simulink model "ad9361_qpsk_test"  (R2019a)
settings: Solver=ode23  StartTime=0.0  StopTime=inf  RelTol=1e-3  EnableMultiTasking=on
undefined symbols (not defined in the file or in its folder): doppler, magnitude
libraries: simulink x11, commdigbbndpm3 x10, dspmathops x4, commrandsrc3 x4, commseqgen3 x4, commfilt2 x3, ad9371_utilities x2, commutil2 x2, ad9361_models x2, commsink2 x1, commchan3 x1, commcnvcod2 x1
settings Model: SimulationMode=accelerator  NumberOfSteps=100  Creator=The MathWorks Inc.  LastModifiedBy=Terasoft
settings SolverCC: MinimalZcImpactIntegration=on
settings DataIOCC: ExternalInput=txWaveform  SaveFormat=StructureWithTime  SaveOutput=off  SignalLogging=off  DSMLogging=off  SaveTime=off  ReturnWorkspaceOutputs=off  OutputSaveName=rx
settings OptimizationCC: DefaultParameterBehavior=Inlined  InlineInvariantSignals=on  EfficientMapNaN2IntZero=off  LifeSpan=inf  SimCompilerOptimization=on
settings DebuggingCC: ReadBeforeWriteMsg=DisableAll  WriteAfterWriteMsg=DisableAll  WriteAfterReadMsg=DisableAll  UnderspecifiedInitializationDetection=Classic  MergeDetectMultiDrivingBlocksExec=none  SolverPrmCheckMsg=warning  InheritedTsInSrcMsg=none  MultiTaskDSMMsg=none  IntegerOverflowMsg=none  AllowSymbolicDim=off  PregeneratedLibrarySubsystemCodeDiagnostic=none  SFUnexpectedBacktrackingDiag=warning  SFNoUnconditionalDefaultTransitionDiag=none  SFUndirectedBroadcastEventsDiag=none  SFExecutionAtInitializationDiag=none  IntegerSaturationMsg=none  ArithmeticOperatorsInVariantConditions=warning
settings HardwareCC: ProdBitPerPointer=32  ProdBitPerSizeT=32  ProdBitPerPtrDiffT=32  ProdLargestAtomicFloat=None  ProdIntDivRoundTo=Undefined  ProdEndianess=Unspecified  ProdWordSize=32  ProdHWDeviceType=32-bit Generic  TargetBitPerPointer=64  TargetBitPerSizeT=64  TargetBitPerPtrDiffT=64  TargetLongLongMode=on  TargetIntDivRoundTo=Zero  TargetEndianess=LittleEndian  TargetWordSize=64  TargetHWDeviceType=MATLAB Host  ProdEqTarget=off
settings ModelReferenceCC: UpdateModelReferenceTargets=IfOutOfDate  PropagateSignalLabelsOutOfModel=off
settings SFSimCC: SFSimEcho=off  SimUseLocalCustomCode=off
settings RTWCC: RTWUseLocalCustomCode=off
settings CodeAppCC: MaxIdLength=128
settings GRTTargetCC: TargetLangStandard=C89/C90 (ANSI)  CombineOutputUpdateFcns=off  GRTInterface=on
settings ConfigComp: CovMetricSettings=dw  CovHtmlReporting=on  CovSaveCumulativeToWorkspaceVar=on  CovSaveSingleToWorkspaceVar=on  CovExternalEMLEnable=off  CovSFcnEnable=off
settings SimscapeCC: ExplicitSolverDiagnosticOptions=none  SimscapeNormalizeSystem=off

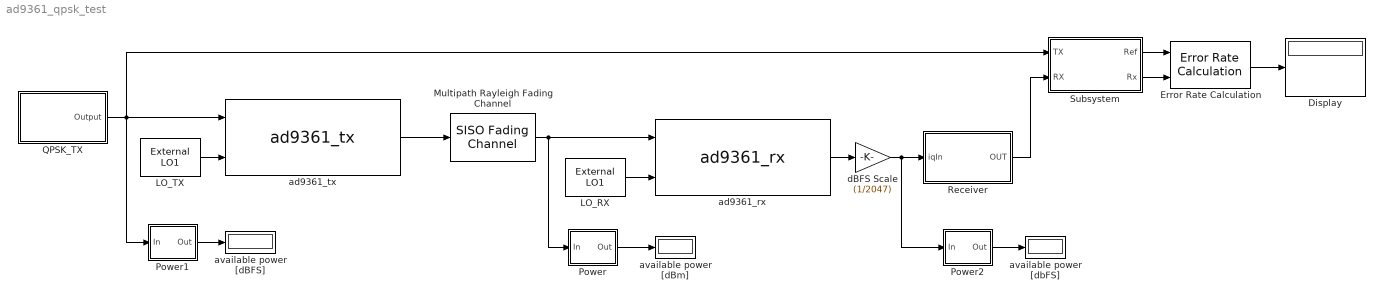
== system ad9361_qpsk_test ==
  Display : Display
  Error Rate Calculation : commsink2/Error Rate Calculation  N=21  st_delay=525  cp_mode=Entire frame  subframe=[]  PMode=Port  WsName=ErrorVec  RsMode2=off  stop=off  numErr=100  maxBits=1e6
      settings: SourceProductName=Communications Toolbox
  LO_RX : ad9371_utilities/External LO1  PN=[-95 -110 -110 -125 -157]  Freq=[1e3 1e4 1e5 1e6 3e6]  PH=Random
      settings: SourceProductName=RF Blockset Models for Analog Devices RF Transceivers  SourceProductBaseCode=SIM_RF_TRANS
  LO_TX : ad9371_utilities/External LO1  PN=[-95 -110 -110 -125 -157]  Freq=[1e3 1e4 1e5 1e6 3e6]  PH=Random
      settings: SourceProductName=RF Blockset Models for Analog Devices RF Transceivers  SourceProductBaseCode=SIM_RF_TRANS
  Multipath Rayleigh Fading Channel : commchan3/SISO Fading Channel  InheritSampleRate=off  SampleRate=122.88e6  PathDelays=[0 3e-8 5e-7]  AveragePathGains=[0 -15 -30]-60 %[0 -15 -30]-40  NormalizePathGains=off  FadingDistribution=Rayleigh  KFactor=3  DirectPathDopplerShift=0  DirectPathInitialPhase=0  MaximumDopplerShift=25  DopplerSpectrum=doppler('Jakes')  ChannelInterpolationMethod=Polyphase  RandomStream=mt19937ar with seed  RandomNumGenerator=shr3cong  Seed=54873  PathGainsOutputPort=off  ChannelFilterDelayOutputPort=off  SimulateUsing=Code generation  Visualization=Off  PathsForDopplerDisplay=1  SamplesToDisplay=25%
      settings: SourceProductName=Communications Toolbox
  Power : Subsystem  mask{R=1}
      mask prompts: R "Reference Impedance [Ohm]"
      mask DialogControl DescGroupVar Prompt: Power Meter
      mask Display: disp('Power \nMeter');
  Power1 : Subsystem  mask{R=1}
      mask prompts: R "Reference Impedance [Ohm]"
      mask DialogControl DescGroupVar Prompt: Power Meter
      mask Display: disp('Power \nMeter');
  Power2 : Subsystem  mask{R=1}
      mask prompts: R "Reference Impedance [Ohm]"
      mask DialogControl DescGroupVar Prompt: Power Meter
      mask Display: disp('Power \nMeter');
  QPSK_TX : Subsystem  mask{Rs=7.68e6, N=4}
      mask prompts: Rs "Sample Rate (Hz)"; N "Samples Per Symbol"
      mask init:
      | PadStart = 100;
      | PadEnd = 100;
      | HeaderBitLength = 16;
      | AGCSequence = 16;
      | AGCPreambleLength = 160;
      | TimingPreambleLength = 28;
      | DFEDataLength = 250;
      | PayloadBitLength = 156;
      | modulatedSymbols = 250;
      | bitsPerSample = 2;
      | 
      | FrameLength = PadStart + AGCPreambleLength + TimingPreambleLength + DFEDataLength + HeaderBitLength + PayloadBitLength + PadEnd;
      | FramePeriod = (FrameLength*N)/Rs;
      mask Display: disp('QPSK Tx')
  Receiver : Subsystem  mask{RadioSampleRate=7.68e6, N=4}
      mask prompts: RadioSampleRate "Sample Rate (Hz)"; N "Samples Per Symbol"
      mask init:
      | numTrainingSamples = 250;
      | VibertiTracebackLength = 34;
      mask Display: disp('QPSK Rx')
  Subsystem : Subsystem  mask{M=4}
      mask prompts: M "Samples per Symbol"
      mask DialogControl DescTextVar Prompt: Ideal QPSK Receiver
      mask Display:
      | disp('Bit Comparison')
      | port_label('input',1,'Tx')
      | port_label('input',2,'Rx')
  ad9361_rx : ad9361_models/ad9361_rx  TestSignal=5MHz LTE  LO=2.4e9  RF=2.4e9  Trf=1/122.88e6  RF_BW=122.88  IQ_rate=7.68
      settings: SourceProductName=RF Blockset Models for Analog Devices RF Transceivers  SourceProductBaseCode=SIM_RF_TRANS
  ad9361_tx : ad9361_models/ad9361_tx  TestSignal=5MHz LTE  LOFreq=2.4e9  Att=0  IQ_rate=7.68  RF_BW=122.88
      settings: SourceProductName=RF Blockset Models for Analog Devices RF Transceivers  SourceProductBaseCode=SIM_RF_TRANS
  available power [dBFS] : Display
  available power [dBm] : Display
  available power [dbFS] : Display
  dBFS Scale : Gain  Gain=(1/2047)
  wires:
  dBFS Scale/1 -> Receiver/1(iqIn), Power2/1(In)
  Power2/1(Out) -> available power [dbFS]/1
  ad9361_rx/1 -> dBFS Scale/1
  Power1/1(Out) -> available power [dBFS]/1
  Power/1(Out) -> available power [dBm]/1
  LO_TX/1 -> ad9361_tx/2
  LO_RX/1 -> ad9361_rx/2
  QPSK_TX/1(Output) -> Subsystem/1(TX), ad9361_tx/1, Power1/1(In)
  Receiver/1(OUT) -> Subsystem/2(RX)
  Error Rate Calculation/1 -> Display/1
  Subsystem/1(Ref) -> Error Rate Calculation/1
  Subsystem/2(Rx) -> Error Rate Calculation/2
  Multipath Rayleigh Fading Channel/1 -> ad9361_rx/1, Power/1(In)
  ad9361_tx/1 -> Multipath Rayleigh Fading Channel/1

== system ad9361_qpsk_test/Power ==
  In : Inport
  CountNCycles : Buffer  N=1024
  Frame Conversion : FrameConversion  OutFrame=Sample-based
  Gain2 : Gain  Gain=1/1024
  Root : Sqrt  SaturateOnIntegerOverflow=on
  Squared : Math  Operator=magnitude^2  SaturateOnIntegerOverflow=on
  Sum : Sum  Inputs=+  CollapseMode=Specified dimension
  dB Conversion : dspmathops/dB Conversion  dBtype=dBm  intype=Amplitude  R=R  fuzz=on
      settings: SourceProductName=DSP System Toolbox
  Out : Outport
  wires:
  dB Conversion/1 -> Out/1
  In/1 -> CountNCycles/1
  Frame Conversion/1 -> dB Conversion/1
  CountNCycles/1 -> Squared/1
  Squared/1 -> Sum/1
  Sum/1 -> Gain2/1
  Root/1 -> Frame Conversion/1
  Gain2/1 -> Root/1

== system ad9361_qpsk_test/Power1 ==
  In : Inport
  CountNCycles : Buffer  N=1024
  Frame Conversion : FrameConversion  OutFrame=Sample-based
  Gain2 : Gain  Gain=1/1024
  Root : Sqrt  SaturateOnIntegerOverflow=on
  Squared : Math  Operator=magnitude^2  SaturateOnIntegerOverflow=on
  Sum : Sum  Inputs=+  CollapseMode=Specified dimension
  dB Conversion : dspmathops/dB Conversion  dBtype=dBm  intype=Amplitude  R=R  fuzz=on
      settings: SourceProductName=DSP System Toolbox
  Out : Outport
  wires:
  Gain2/1 -> Root/1
  Root/1 -> Frame Conversion/1
  Sum/1 -> Gain2/1
  Squared/1 -> Sum/1
  CountNCycles/1 -> Squared/1
  Frame Conversion/1 -> dB Conversion/1
  In/1 -> CountNCycles/1
  dB Conversion/1 -> Out/1

== system ad9361_qpsk_test/Power2 ==
  In : Inport
  CountNCycles : Buffer  N=1024
  Frame Conversion : FrameConversion  OutFrame=Sample-based
  Gain2 : Gain  Gain=1/1024
  Root : Sqrt  SaturateOnIntegerOverflow=on
  Squared : Math  Operator=magnitude^2  SaturateOnIntegerOverflow=on
  Sum : Sum  Inputs=+  CollapseMode=Specified dimension
  dB Conversion : dspmathops/dB Conversion  dBtype=dB  intype=Amplitude  R=R  fuzz=on
      settings: SourceProductName=DSP System Toolbox
  Out : Outport
  wires:
  Gain2/1 -> Root/1
  Root/1 -> Frame Conversion/1
  Sum/1 -> Gain2/1
  Squared/1 -> Sum/1
  CountNCycles/1 -> Squared/1
  Frame Conversion/1 -> dB Conversion/1
  In/1 -> CountNCycles/1
  dB Conversion/1 -> Out/1

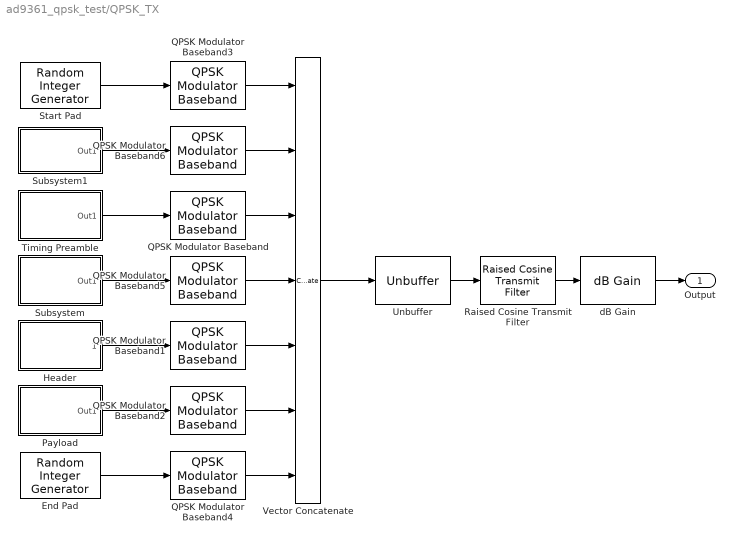
== system ad9361_qpsk_test/QPSK_TX ==
  End Pad : commrandsrc3/Random Integer Generator  SetSize=4  SeedSource=Parameter  Seed=984154  SampleTime=FramePeriod/PadEnd  SamplesPerFrame=PadEnd  OutputDataType=double  SimulateUsing=Interpreted execution
      settings: SourceProductName=Communications Toolbox
  Header : Subsystem  mask{HeaderLen=16, HeaderData=[0 0 0 1 1 1 0 0 1 0 0 0 0 0 0 0 ].'}
      mask prompts: HeaderLen "Number of Header Bits"; HeaderData "Header Data Bits"
      mask DialogControl DescTextVar Prompt: Header Bit Generation
      mask Display: disp(['Header' char(10) 'Bit' char(10) 'Generation']);
  Payload : Subsystem  mask{nPayloadSymbols=16, rate=1/2, M=4, tbl=34}
      mask prompts: nPayloadSymbols "Number of Payload Symbols"; rate "Coding Bit Rate"; M "Modulation (4 for QPSK)"; tbl "Viterbi Traceback Length"
      mask DialogControl DescTextVar Prompt: Payload Bit Generation
      mask Display: disp(['Payload' char(10) 'Bit' char(10) 'Generation']);
  QPSK Modulator Baseband{,3..4,6} (4 alike) : commdigbbndpm3/QPSK Modulator Baseband  InType=Integer  Enc=Binary  Ph=pi/4  outDtype=double  outWordLen=16  outUDDataType=sfix(16)  outFracLenMode=Best precision  outFracLen=15  outDataTypeStr=double  outLastDataTypeStr=double
      settings: SourceProductName=Communications Toolbox
  QPSK Modulator Baseband1 : commdigbbndpm3/QPSK Modulator Baseband  InType=Bit  Enc=Binary  Ph=pi/4  outDtype=double  outWordLen=16  outUDDataType=sfix(16)  outFracLenMode=Best precision  outFracLen=15  outDataTypeStr=double  outLastDataTypeStr=double
      settings: SourceProductName=Communications Toolbox
  QPSK Modulator Baseband2 : commdigbbndpm3/QPSK Modulator Baseband  InType=Bit  Enc=Binary  Ph=pi/4  outDtype=double  outWordLen=16  outUDDataType=sfix(16)  outFracLenMode=Best precision  outFracLen=15  outDataTypeStr=double  outLastDataTypeStr=double
      settings: SourceProductName=Communications Toolbox
  QPSK Modulator Baseband5 : commdigbbndpm3/QPSK Modulator Baseband  InType=Bit  Enc=Binary  Ph=pi/4  outDtype=double  outWordLen=16  outUDDataType=sfix(16)  outFracLenMode=Best precision  outFracLen=15  outDataTypeStr=double  outLastDataTypeStr=double
      settings: SourceProductName=Communications Toolbox
  Raised Cosine Transmit Filter : commfilt2/Raised Cosine Transmit Filter  filtType=Square root  R=0.5  filtSpan=8  N=N  filterGain=1  RateOptions=Allow multirate processing  framing=Mute  checkCoeff=off  variableName=rcTxFilt  checkGain=Normalized  sampMode=Mute  saveAsFlag=0  currentFiltSpan=8  D=(8)/2  launchFVT=on  roundingMode=Floor  overflowMode=off  coeffDataTypeStr=Inherit: Same word length as input  coeffMin=[]  coeffMax=[]  coeffLastDataTypeStr=Inherit: Same word length as input  outputDataTypeStr=Inherit: Same as accumulator  outputMin=[]  outputMax=[]  outputLastDataTypeStr=Inherit: Same as accumulator
      settings: SourceProductName=Communications Toolbox
  Start Pad : commrandsrc3/Random Integer Generator  SetSize=4  SeedSource=Parameter  Seed=123456  SampleTime=FramePeriod/PadStart  SamplesPerFrame=PadStart  OutputDataType=double  SimulateUsing=Interpreted execution
      settings: SourceProductName=Communications Toolbox
  Subsystem : Subsystem
      mask Display: disp('DFE Training')
  Subsystem1 : Subsystem
      mask Display: disp('AGC Preamble')
  Timing Preamble : Subsystem
      mask Display: disp('Timing Preamble')
  Unbuffer : Unbuffer
  Vector Concatenate : Concatenate  NumInputs=7
  dB Gain : dspmathops/dB Gain  dB=-24  intype=Amplitude
      settings: SourceProductName=DSP System Toolbox  SourceProductBaseCode=DS
  Output : Outport
  wires:
  QPSK Modulator Baseband3/1 -> Vector Concatenate/1
  Start Pad/1 -> QPSK Modulator Baseband3/1
  Payload/1("Out1 ") -> QPSK Modulator Baseband2/1
  Timing Preamble/1(Out1) -> QPSK Modulator Baseband/1
  Header/1(" ") -> QPSK Modulator Baseband1/1
  End Pad/1 -> QPSK Modulator Baseband4/1
  Vector Concatenate/1 -> Unbuffer/1
  Unbuffer/1 -> Raised Cosine Transmit Filter/1
  Raised Cosine Transmit Filter/1 -> dB Gain/1
  dB Gain/1 -> Output/1
  Subsystem/1(Out1) -> QPSK Modulator Baseband5/1
  QPSK Modulator Baseband/1 -> Vector Concatenate/3
  QPSK Modulator Baseband5/1 -> Vector Concatenate/4
  QPSK Modulator Baseband1/1 -> Vector Concatenate/5
  QPSK Modulator Baseband2/1 -> Vector Concatenate/6
  QPSK Modulator Baseband4/1 -> Vector Concatenate/7
  QPSK Modulator Baseband6/1 -> Vector Concatenate/2
  Subsystem1/1(Out1) -> QPSK Modulator Baseband6/1

== system ad9361_qpsk_test/Receiver ==
  iqIn : Inport
  Downsample : DownSample  N=N  RateOptions=Allow multirate processing
  Frame Recover : Subsystem
  Gardner Timing Recovery : Subsystem
  QPSK Demodulator Baseband : commdigbbndpm3/QPSK Demodulator Baseband  OutType=Integer  DecType=Hard decision  VarSource=Dialog  Variance=1  Dec=Binary  Ph=pi/4  outDtype1=boolean  outDtype2=Inherit via internal rule  derotateFactorWordLen=16  derotateFactorDataTypeStr=Inherit: Same word length as input  derotateFactorLastDataTypeStr=Inherit: Same word length as input
      settings: SourceProductName=Communications Toolbox
  Raised Cosine Receive Filter : commfilt2/Raised Cosine Receive Filter  filtType=Square root  R=0.5  filtSpan=8  N=N  downFactor=1  downOffset=0  filterGain=1  RateOptions=Allow multirate processing  framing=Mute  checkCoeff=off  variableName=rcRxFilt  currentFiltSpan=8  D=(8)/2  inputOffset=0  sampMode=Mute  saveAsFlag=0  rateMode=Downsampling  checkGain=Normalized  launchFVT=on  roundingMode=Floor  overflowMode=off  coeffDataTypeStr=Inherit: Same word length as input  coeffMin=[]  coeffMax=[]  coeffLastDataTypeStr=Inherit: Same word length as input  accumDataTypeStr=Inherit: Same as product output  accumLastDataTypeStr=Inherit: Same as product output  outputDataTypeStr=Inherit: Same as accumulator  outputMin=[]  outputMax=[]  outputLastDataTypeStr=Inherit: Same as accumulator
      settings: SourceProductName=Communications Toolbox
  Zero-Order Hold2 : ZeroOrderHold  SampleTime=1/RadioSampleRate
  OUT : Outport
  wires:
  iqIn/1 -> Raised Cosine Receive Filter/1
  QPSK Demodulator Baseband/1 -> Zero-Order Hold2/1
  Frame Recover/1(Out) -> QPSK Demodulator Baseband/1
  Gardner Timing Recovery/2(Out) -> Frame Recover/1(In)
  Raised Cosine Receive Filter/1 -> Gardner Timing Recovery/1(In)
  Zero-Order Hold2/1 -> Downsample/1
  Downsample/1 -> OUT/1
  Gardner Timing Recovery/1(strobe) -> Frame Recover/Enable

== system ad9361_qpsk_test/Subsystem ==
  TX : Inport
  RX : Inport  Port=2
  Display1 : Display
  Display2 : Display
  Find Delay : commutil2/Find Delay  corrLength=226  chgSigOP=on  stopUpdate=off  numConstDelay=3
      settings: SourceProductName=Communications Toolbox  SourceProductBaseCode=CM
  QPSK Demodulator Baseband : commdigbbndpm3/QPSK Demodulator Baseband  OutType=Integer  DecType=Hard decision  VarSource=Dialog  Variance=1  Dec=Binary  Ph=pi/4  outDtype1=boolean  outDtype2=Inherit via internal rule  derotateFactorWordLen=16  derotateFactorDataTypeStr=Inherit: Same word length as input  derotateFactorLastDataTypeStr=Inherit: Same word length as input
      settings: SourceProductName=Communications Toolbox
  Raised Cosine Receive Filter : commfilt2/Raised Cosine Receive Filter  filtType=Square root  R=0.5  filtSpan=8  N=M  downFactor=M  downOffset=0  filterGain=1  RateOptions=Allow multirate processing  framing=Mute  checkCoeff=off  variableName=rcRxFilt1  currentFiltSpan=2*M  D=(2*M)/2  inputOffset=0  sampMode=Mute  saveAsFlag=0  rateMode=Downsampling  checkGain=Normalized  launchFVT=on  roundingMode=Floor  overflowMode=off  coeffDataTypeStr=Inherit: Same word length as input  coeffMin=[]  coeffMax=[]  coeffLastDataTypeStr=Inherit: Same word length as input  accumDataTypeStr=Inherit: Same as product output  accumLastDataTypeStr=Inherit: Same as product output  outputDataTypeStr=Inherit: Same as accumulator  outputMin=[]  outputMax=[]  outputLastDataTypeStr=Inherit: Same as accumulator
      settings: SourceProductName=Communications Toolbox
  Time Scope : Scope  Commented=on  NumInputPorts=2
  Ref : Outport
  Rx : Outport  Port=2
  wires:
  Raised Cosine Receive Filter/1 -> QPSK Demodulator Baseband/1
  TX/1 -> Raised Cosine Receive Filter/1
  Find Delay/1 -> Display1/1
  QPSK Demodulator Baseband/1 -> Ref/1, Time Scope/1, Find Delay/1
  Find Delay/2 -> Display2/1
  RX/1 -> Time Scope/2, Find Delay/2, Rx/1

== system ad9361_qpsk_test/QPSK_TX/Header ==
  Constant2 : Constant  Value=[HeaderData ~HeaderData].'  SampleTime=FramePeriod
  Reshape : Reshape  OutputDimensionality=Customize  OutputDimensions=[HeaderLen*2,1]
  " " : Outport
  wires:
  Constant2/1 -> Reshape/1
  Reshape/1 -> " "/1

== system ad9361_qpsk_test/QPSK_TX/Payload ==
  Constant : Constant  Value=[1 0 1 1 0 0 1 1 1 1 1 0 1 1 0 0 1 1 1 1 1 0 1 1 0 0 1 1 1 1 1 0 1 1 0 0 1 1 1 1].'  SampleTime=FramePeriod
  Convolutional Encoder : commcnvcod2/Convolutional Encoder  trellis=poly2trellis(7, [171 133])  opMode=Continuous  DelayedResetAction=off  hasIniStPort=off  hasFinStPort=off  usePuncVector=off  punctureVector=[1; 1; 0; 1; 0; 1]  reset=Unused parameter value
      settings: SourceProductName=Communications Toolbox  SourceProductBaseCode=CM
  General CRC Generator : commcrc2/General CRC Generator  genPoly='z^32 + z^26 + z^23 + z^22 + z^16 + z^12 + z^11 + z^10 + z^8 + z^7 + z^5 + z^4 + z^2 + z + 1'  iniStates=0  directMethod=off  reflectInputBytes=off  reflectChecksums=off  finalXOR=0  numChecksums=1
      settings: SourceProductName=Communications Toolbox  SourceProductBaseCode=CM
  Matrix Concatenate : Concatenate  NumInputs=3  Mode=Multidimensional array
  Scrambler : commsequence2/Scrambler  M=2  poly='1 + z^-1 + z^-3 + z^-5+ z^-7'  iniStaSource=Dialog Parameter  ini_sta=[0 1 0 0 0 1 0]  resetViaPort=off
      settings: SourceProductName=Communications Toolbox  SourceProductBaseCode=CM
  lagBits : commrandsrc3/Random Integer Generator  SetSize=2  SeedSource=Parameter  Seed=9864  SampleTime=FramePeriod/(tbl/rate)  SamplesPerFrame=tbl/rate  OutputDataType=double  SimulateUsing=Interpreted execution
      settings: SourceProductName=Communications Toolbox
  txData : commrandsrc3/Random Integer Generator  SetSize=2  SeedSource=Parameter  Seed=5689  SampleTime=FramePeriod/(nPayloadSymbols*log2(M)*rate)  SamplesPerFrame=nPayloadSymbols*log2(M)*rate  OutputDataType=double  SimulateUsing=Interpreted execution
      settings: SourceProductName=Communications Toolbox
  "Out1 " : Outport
  wires:
  Constant/1 -> Matrix Concatenate/2
  txData/1 -> General CRC Generator/1
  Scrambler/1 -> Convolutional Encoder/1
  General CRC Generator/1 -> Matrix Concatenate/1
  lagBits/1 -> Matrix Concatenate/3
  Convolutional Encoder/1 -> "Out1 "/1
  Matrix Concatenate/1 -> Scrambler/1

== system ad9361_qpsk_test/QPSK_TX/Subsystem ==
  PN Sequence Generator : commseqgen3/PN Sequence Generator  poly='z^5 + z^3 + z^1 + 1'  ini_sta=[1 1 1 0 0]  outBitMaskSource=Dialog parameter  shift=0  outVarSiz=off  maxOutSizeMode=Dialog parameter  maxOutSize=[10 1]  Ts=FramePeriod/DFEDataLength  sampPerFrame=modulatedSymbols*bitsPerSample  reset=off  bitPackedOutputs=off  outDataType=double  numPackedBits=8  bitPackDataSigned=off  bitPackedOutDType=double
      settings: SourceProductName=Communications Toolbox
  Out1 : Outport
  wires:
  PN Sequence Generator/1 -> Out1/1

== system ad9361_qpsk_test/QPSK_TX/Subsystem1 ==
  Barker Code Generator : commseqgen3/Barker Code Generator  Length=7  LengthSimulink=13  SampleTime=FramePeriod/AGCSequence  SamplesPerFrame=AGCSequence  OutputDataType=double  SimulateUsing=Code generation
      settings: SourceProductName=Communications Toolbox  SourceProductBaseCode=CM
  Bias : Bias  Bias=1
  One : Constant  Value=ones(1,10)  VectorParams1D=off  OutDataTypeStr=Inherit: Inherit via back propagation  SampleTime=-1
  Product : Product  Multiplication=Matrix(*)
  Reshape : Reshape  OutputDimensionality=Column vector (2-D)
  Out1 : Outport
  wires:
  Barker Code Generator/1 -> Bias/1
  Bias/1 -> Product/1
  Product/1 -> Reshape/1
  One/1 -> Product/2
  Reshape/1 -> Out1/1

== system ad9361_qpsk_test/QPSK_TX/Timing Preamble ==
  Add Constant : Bias  Bias=1
  Timing Preamble : commseqgen3/Barker Code Generator  Length=7  LengthSimulink=11  SampleTime=FramePeriod/TimingPreambleLength  SamplesPerFrame=TimingPreambleLength  OutputDataType=double  SimulateUsing=Code generation
      settings: SourceProductName=Communications Toolbox  SourceProductBaseCode=CM
  Out1 : Outport
  wires:
  Timing Preamble/1 -> Add Constant/1
  Add Constant/1 -> Out1/1

== system ad9361_qpsk_test/Receiver/Frame Recover ==
  In : Inport
  Enable : EnablePort
  Barker Locate : Subsystem  mask{Threshold=1.2}
      mask init:
      | barker = comm.BarkerCode('SamplesPerFrame', 28, 'Length', 11);
      | seq = barker()+1;
      | M = 4;
      | hPSKModTrain   = comm.PSKModulator(M, ...
      |     'PhaseOffset',pi/4, ...
      |     'SymbolMapping','Binary');
      | xPreambleSeq = hPSKModTrain(seq);
  DFE : Subsystem
  Frequency Recovery : Subsystem
  Rx Constellation : ConstellationDiagram
  Out : Outport
  wires:
  DFE/1(Out) -> Out/1, Rx Constellation/1
  Frequency Recovery/1(Out) -> Barker Locate/1(In)
  In/1 -> Frequency Recovery/1(In)
  Barker Locate/1(Out) -> DFE/1(In)
  Barker Locate/2(Detector) -> DFE/2(Trigger)

== system ad9361_qpsk_test/Receiver/Gardner Timing Recovery ==
  In : Inport
  Delay : Delay  DelayLength=1
  Delay1 : Delay  DelayLength=1
  Gardner TED Blocks : Subsystem
  InterpControl_Blocks : Subsystem
  Interpolator : Subsystem
  LoopFilter : Subsystem  mask{zeta=sqrt(2), BnTs=0.01, Kp=2.7, SPS=N}
      mask prompts: zeta "DampingFactor"; BnTs "NormalizedLoopBandwidth"; Kp "DetectionGain"; SPS "Samples Per Symbol"
      mask init:
      | K0 = -1;
      | theta = BnTs/SPS/(zeta + 0.25/zeta);
      | d  = (1 + 2*zeta*theta + theta^2) * K0 * Kp;
      | ProportionalGain = (4*zeta*theta) /d;
      | IntegratorGain   = (4*theta*theta)/d;
  strobe : Outport  InitialOutput=false
  Out : Outport  Port=2  InitialOutput=0
  wires:
  In/1 -> Interpolator/1(In1)
  LoopFilter/1(v) -> InterpControl_Blocks/1(e)
  InterpControl_Blocks/2(mu) -> Delay/1
  InterpControl_Blocks/1(strobe) -> Delay1/1
  Gardner TED Blocks/1(e) -> LoopFilter/1(e)
  Interpolator/1(Out1) -> Out/1, Gardner TED Blocks/1(data)
  Delay1/1 -> strobe/1, Gardner TED Blocks/2(strobe)
  Delay/1 -> Interpolator/2(mu)

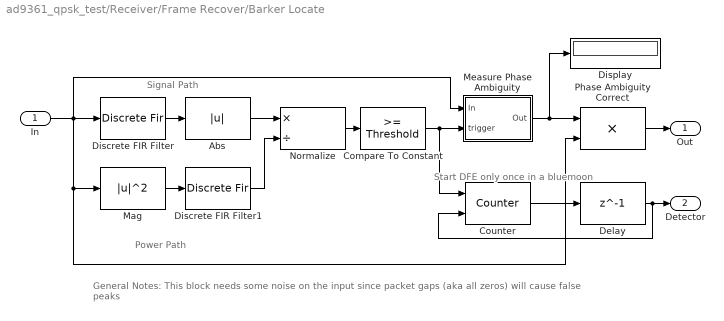
== system ad9361_qpsk_test/Receiver/Frame Recover/Barker Locate ==
  note: Start DFE only once in a bluemoon
  note: General Notes:
      | This block needs some noise on the input since packet gaps (aka all zeros) will cause false peaks
  note: Power Path
  note: Signal Path
  In : Inport
  Abs : Abs
  Compare To Constant : simulink/Logic and Bit Operations/Compare To Constant  relop=>=  const=Threshold  OutDataTypeStr=boolean
  Counter : dspswit3/Counter  Direction=Up  CountEvent=Rising edge  CounterSize=User defined  MaxCount=100  InitialCount=0  Output=Hit  HitValue=100  ResetInput=on  SamplesPerFrame=1  Ts=1  CntDtype=double  HitDtype=Logical
  Delay : Delay  DelayLength=1  InitialCondition=1
  Discrete FIR Filter : DiscreteFir  Coefficients=xPreambleSeq(end:-1:1).'  AccumDataTypeStr=Inherit: Same as product output  OutDataTypeStr=Inherit: Same as input
  Discrete FIR Filter1 : DiscreteFir  Coefficients=ones(1,length(xPreambleSeq)*1)/1  InitialStates=1  AccumDataTypeStr=Inherit: Same as product output  OutDataTypeStr=Inherit: Same as input
  Display : Display
  Mag : Math  Operator=magnitude^2  SaturateOnIntegerOverflow=on
  Measure Phase Ambiguity : Subsystem
  Normalize : Product  Inputs=*/
  Phase Ambiguity Correct : Product
  Out : Outport
  Detector : Outport  Port=2
  wires:
  Discrete FIR Filter/1 -> Abs/1
  Abs/1 -> Normalize/1
  Normalize/1 -> Compare To Constant/1
  Phase Ambiguity Correct/1 -> Out/1
  Discrete FIR Filter1/1 -> Normalize/2
  Mag/1 -> Discrete FIR Filter1/1
  In/1 -> Discrete FIR Filter/1, Measure Phase Ambiguity/1(In), Mag/1, Phase Ambiguity Correct/2
  Measure Phase Ambiguity/1(Out) -> Display/1, Phase Ambiguity Correct/1
  Compare To Constant/1 -> Measure Phase Ambiguity/2(trigger), Counter/1
  Counter/1 -> Delay/1
  Delay/1 -> Counter/2, Detector/1

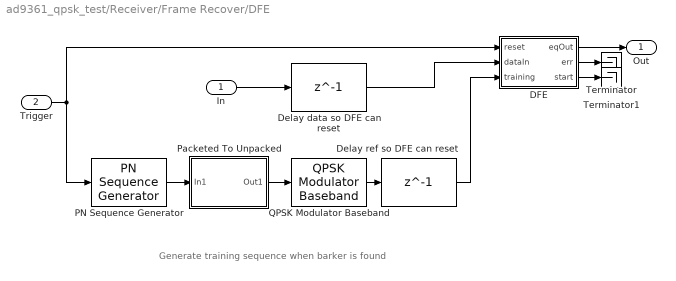
== system ad9361_qpsk_test/Receiver/Frame Recover/DFE ==
  note: Generate training sequence when barker is found
  In : Inport  PortDimensions=1
  Trigger : Inport  Port=2
  DFE : Subsystem  mask{numFTaps=6, numBTaps=3, mu=0.01, refTap=2+1}
      mask prompts: numFTaps "Num Forward Taps"; numBTaps "Num Backward Taps"; mu "Step Size"; refTap "Reference Tap"
  Delay data so DFE can reset : Delay  DelayLength=1
  Delay ref so DFE can reset : Delay  DelayLength=1
  PN Sequence Generator : commseqgen3/PN Sequence Generator  poly='z^5 + z^3 + z^1 + 1'  ini_sta=[1 1 1 0 0]  outBitMaskSource=Dialog parameter  shift=0  outVarSiz=off  maxOutSizeMode=Dialog parameter  maxOutSize=[10 1]  Ts=-1  sampPerFrame=1  reset=on  bitPackedOutputs=on  outDataType=Smallest unsigned integer  numPackedBits=2  bitPackDataSigned=off  bitPackedOutDType=Smallest integer
      settings: SourceProductName=Communications Toolbox
  Packeted To Unpacked : Subsystem
  QPSK Modulator Baseband : commdigbbndpm3/QPSK Modulator Baseband  InType=Bit  Enc=Binary  Ph=pi/4  outDtype=double  outWordLen=16  outUDDataType=sfix(16)  outFracLenMode=User-defined  outFracLen=14  outDataTypeStr=double  outLastDataTypeStr=double
      settings: SourceProductName=Communications Toolbox
  Terminator : Terminator
  Terminator1 : Terminator
  Out : Outport
  wires:
  In/1 -> Delay data so DFE can reset/1
  PN Sequence Generator/1 -> Packeted To Unpacked/1(In1)
  Packeted To Unpacked/1(Out1) -> QPSK Modulator Baseband/1
  QPSK Modulator Baseband/1 -> Delay ref so DFE can reset/1
  DFE/2(err) -> Terminator/1
  Delay ref so DFE can reset/1 -> DFE/3(training)
  Delay data so DFE can reset/1 -> DFE/2(dataIn)
  Trigger/1 -> DFE/1(reset), PN Sequence Generator/1
  DFE/1(eqOut) -> Out/1
  DFE/3(start) -> Terminator1/1

== system ad9361_qpsk_test/Receiver/Frame Recover/Frequency Recovery ==
  note: Max Phase Lock Delay= 1.3/(NormLoopBandwidth*SampleRate)
  note: Frequency Lock Delay = SampleRate*4*NormalizedPullInRange^2)/ (SampleRate*NormLoopBandwidth)^3;
  note: Pull in range (Hz) = 2*pi*sqrt(2)*DampingFactor*NormLoopBandwidth*SampleRate
  In : Inport
  Delay : Delay  DelayLength=1
  Loop Filter : Subsystem  mask{BnTs=0.01, zeta=N*1/sqrt(2), N=1}
      mask prompts: BnTs "Normalized Loop Bandwidth"; zeta "Damping Factor"; N "Number of Samples/Symbol"
      mask init:
      | % See C.57 to C.61 in Michael Rice's "Digital Communications 
      | % - A Discrete-Time Approach" for details
      | 
      | %theta = BnTs/(zeta+0.25/zeta);  %0.0385
      | %d = 1 + 2*zeta*theta + theta*theta; %1.1938
      | %K1 = zeta*theta/d; %0.0805
      | %K2 = theta*theta/(d*2); %6.1958e-04
      | 
      | %%
      | DampingFactor = zeta;
      | samplesPerSymbol = N;
      | NormalizedLoopBandwidth = BnTs;
      | %
      | PhaseRecoveryLoopBandwidth = NormalizedLoopBandwidth*samplesPerSymbol;
      |  
      | PhaseRecoveryGain = samplesPerSymbol;
      |  
      | PhaseErrorDetectorGain = 1;
      | 
      | 
      | theta = PhaseRecoveryLoopBandwidth/...
      |     ((DampingFactor + 0.25/DampingFactor)*samplesPerSymbol);
      |  
      | d = 1 + 2*DampingFactor*theta + theta*theta;
      |  
      | % K1
      | K1 = (4*DampingFactor*theta/d)/...
      |     (PhaseErrorDetectorGain*PhaseRecoveryGain);
      | % K2
      | K2 = (4/samplesPerSymbol*theta*theta/d)/...
      |     (PhaseErrorDetectorGain*PhaseRecoveryGain);
      mask Display: disp('Loop Filter')
  PED : MATLAB Function  TreatAsAtomicUnit=on
  Phase Shift FP : Subsystem
  Out : Outport
  wires:
  Loop Filter/1(v) -> Phase Shift FP/2(Phi)
  Delay/1 -> PED/1(In), Out/1
  PED/1(e) -> Loop Filter/1(e)
  In/1 -> Phase Shift FP/1(In1)
  Phase Shift FP/1(Out1) -> Delay/1

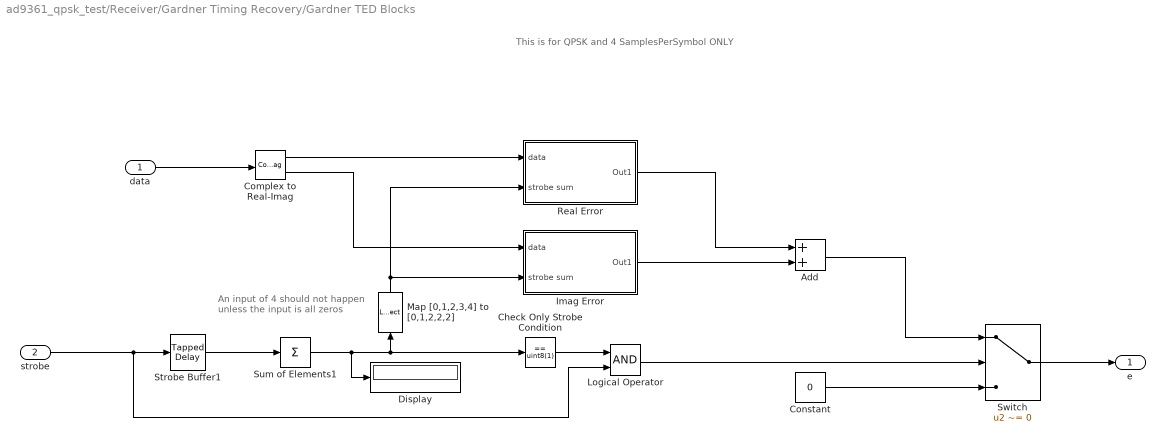
== system ad9361_qpsk_test/Receiver/Gardner Timing Recovery/Gardner TED Blocks ==
  note: This is for QPSK and 4 SamplesPerSymbol ONLY
  note: An input of 4 should not
      | happen unless the input is all zeros
  data : Inport
  strobe : Inport  Port=2
  Add : Sum  OutDataTypeStr=Inherit: Inherit via back propagation
  Check Only Strobe Condition : simulink/Logic and Bit Operations/Compare To Constant  relop===  const=uint8(1)  OutDataTypeStr=boolean
  Complex to Real-Imag : ComplexToRealImag
  Constant : Constant  Value=0  SampleTime=-1
  Display : Display
  Imag Error : Subsystem
  Logical Operator : Logic  AllPortsSameDT=off  OutDataTypeStr=boolean
  Map [0,1,2,3,4] to [0,1,2,2,2] : LookupNDDirect  NumberOfTableDimensions=1  Table=[0 1 2 2 2]  DiagnosticForOutOfRangeInput=Error  TableDataTypeStr=uint8
  Real Error : Subsystem
  Strobe Buffer1 : simulink/Discrete/Tapped Delay  vinit=0.0  samptime=-1  NumDelays=N-1  DelayOrder=Oldest  includeCurrent=on
  Sum of Elements1 : Sum  Inputs=+  OutDataTypeStr=int8
  Switch : Switch  Criteria=u2 ~= 0  OutDataTypeStr=Inherit: Inherit via back propagation  SaturateOnIntegerOverflow=on
  e : Outport
  wires:
  Logical Operator/1 -> Switch/2
  Add/1 -> Switch/1
  Strobe Buffer1/1 -> Sum of Elements1/1
  Map [0,1,2,3,4] to [0,1,2,2,2]/1 -> Real Error/2(strobe sum), Imag Error/2(strobe sum)
  data/1 -> Complex to Real-Imag/1
  Complex to Real-Imag/1 -> Real Error/1(data)
  Check Only Strobe Condition/1 -> Logical Operator/1
  Sum of Elements1/1 -> Map [0,1,2,3,4] to [0,1,2,2,2]/1, Check Only Strobe Condition/1, Display/1
  Complex to Real-Imag/2 -> Imag Error/1(data)
  Switch/1 -> e/1
  Real Error/1(Out1) -> Add/1
  Imag Error/1(Out1) -> Add/2
  Constant/1 -> Switch/3
  strobe/1 -> Logical Operator/2, Strobe Buffer1/1

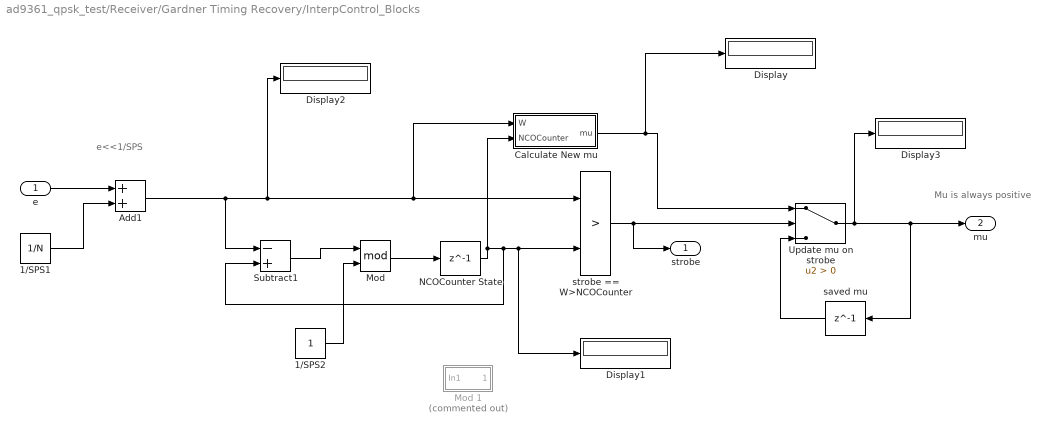
== system ad9361_qpsk_test/Receiver/Gardner Timing Recovery/InterpControl_Blocks ==
  note: Mu is always positive
  note: e<<1/SPS
  e : Inport
  1/SPS1 : Constant  Value=1/N  SampleTime=-1
  1/SPS2 : Constant  SampleTime=-1
  Add1 : Sum  OutDataTypeStr=Inherit: Inherit via back propagation
  Calculate New mu : Subsystem
  Display{,1..3} (4 alike) : Display
  Mod : Math  Operator=mod  SaturateOnIntegerOverflow=on
  Mod 1 : Subsystem  Commented=on
  NCOCounter State : Delay  DelayLength=1  InitialCondition=0
  Subtract1 : Sum  Inputs=-+  OutDataTypeStr=Inherit: Same as first input
  Update mu on strobe : Switch  Criteria=u2 > Threshold
  saved mu : Delay  DelayLength=1
  strobe == W>NCOCounter : RelationalOperator  Operator=>  OutDataTypeStr=boolean  RndMeth=Nearest
  strobe : Outport
  mu : Outport  Port=2
  wires:
  1/SPS2/1 -> Mod/2
  Add1/1 -> Subtract1/1, Display2/1, strobe == W>NCOCounter/1, Calculate New mu/1(W)
  1/SPS1/1 -> Add1/2
  Mod/1 -> NCOCounter State/1
  Subtract1/1 -> Mod/1
  NCOCounter State/1 -> Calculate New mu/2(NCOCounter), strobe == W>NCOCounter/2, Display1/1, Subtract1/2
  e/1 -> Add1/1
  Calculate New mu/1(mu) -> Update mu on strobe/1, Display/1
  saved mu/1 -> Update mu on strobe/3
  Update mu on strobe/1 -> saved mu/1, mu/1, Display3/1
  strobe == W>NCOCounter/1 -> strobe/1, Update mu on strobe/2

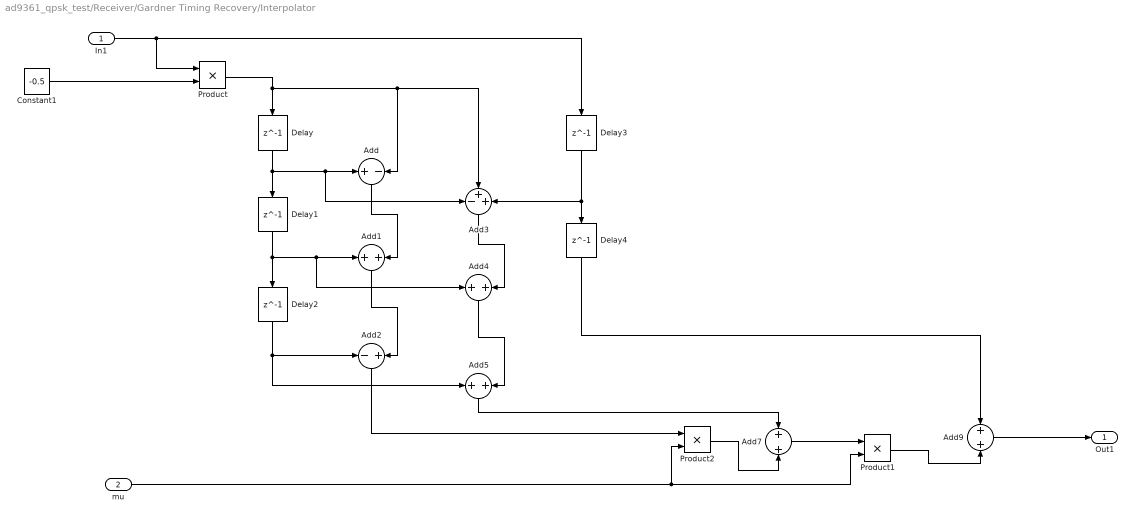
== system ad9361_qpsk_test/Receiver/Gardner Timing Recovery/Interpolator ==
  In1 : Inport
  mu : Inport  Port=2
  Add : Sum  Inputs=+-  OutDataTypeStr=Inherit: Same as first input
  Add{1,4..5,7,9} (5 alike) : Sum
  Add2 : Sum  Inputs=-+
  Add3 : Sum  Inputs=-++
  Constant1 : Constant  Value=-0.5  OutDataTypeStr=double  SampleTime=-1
  Delay{,1..4} (5 alike) : Delay  DelayLength=1
  Product : Product  OutDataTypeStr=double
  Product1 : Product
  Product2 : Product
  Out1 : Outport
  wires:
  Add9/1 -> Out1/1
  mu/1 -> Product2/2, Product1/2
  Add7/1 -> Product1/1
  Delay4/1 -> Add9/1
  Add2/1 -> Product2/1
  Add5/1 -> Add7/1
  Product1/1 -> Add9/2
  Delay3/1 -> Add3/3, Delay4/1
  Product2/1 -> Add7/2
  Add4/1 -> Add5/2
  Add3/1 -> Add4/2
  Add1/1 -> Add2/2
  Delay2/1 -> Add2/1, Add5/1
  Add/1 -> Add1/2
  Delay1/1 -> Delay2/1, Add1/1, Add4/1
  Delay/1 -> Delay1/1, Add/1, Add3/1
  Product/1 -> Delay/1, Add/2, Add3/2
  In1/1 -> Product/1, Delay3/1
  Constant1/1 -> Product/2

== system ad9361_qpsk_test/Receiver/Gardner Timing Recovery/LoopFilter ==
  e : Inport
  Add : Sum
  Add1 : Sum
  Delay : Delay  DelayLength=1
  Delay1 : Delay  DelayLength=1
  Intergrator Gain : Gain  Gain=IntegratorGain
  Proportional Gain : Gain  Gain=ProportionalGain
  v : Outport
  wires:
  Proportional Gain/1 -> Add1/2
  Add1/1 -> v/1
  Delay1/1 -> Add/2
  Delay/1 -> Add/1
  Intergrator Gain/1 -> Delay/1
  e/1 -> Intergrator Gain/1, Proportional Gain/1
  Add/1 -> Delay1/1, Add1/1

== system ad9361_qpsk_test/Receiver/Frame Recover/Barker Locate/Measure Phase Ambiguity ==
  In : Inport
  trigger : Inport  Port=2
  Discrete FIR Filter1 : DiscreteFir  Coefficients=exp(-j*pi/2).*xPreambleSeq(end:-1:1).'  InputProcessing=Columns as channels (frame based)  AccumDataTypeStr=Inherit: Same as product output  OutDataTypeStr=Inherit: Same as input
  Discrete FIR Filter2 : DiscreteFir  Coefficients=xPreambleSeq(end:-1:1).'  InputProcessing=Columns as channels (frame based)  AccumDataTypeStr=Inherit: Same as product output  OutDataTypeStr=Inherit: Same as input
  Discrete FIR Filter3 : DiscreteFir  Coefficients=exp(-j*pi).*xPreambleSeq(end:-1:1).'  InputProcessing=Columns as channels (frame based)  AccumDataTypeStr=Inherit: Same as product output  OutDataTypeStr=Inherit: Same as input
  Discrete FIR Filter4 : DiscreteFir  Coefficients=exp(-j*pi*3/2).*xPreambleSeq(end:-1:1).'  InputProcessing=Columns as channels (frame based)  AccumDataTypeStr=Inherit: Same as product output  OutDataTypeStr=Inherit: Same as input
  Find Max and Set Output Shift : Subsystem
  Out : Outport
  wires:
  Find Max and Set Output Shift/1(Out1) -> Out/1
  In/1 -> Discrete FIR Filter4/1, Discrete FIR Filter3/1, Discrete FIR Filter1/1, Discrete FIR Filter2/1
  Discrete FIR Filter2/1 -> Find Max and Set Output Shift/1(In1)
  Discrete FIR Filter1/1 -> Find Max and Set Output Shift/2(In2)
  Discrete FIR Filter3/1 -> Find Max and Set Output Shift/3(In)
  Discrete FIR Filter4/1 -> Find Max and Set Output Shift/4(In5)
  trigger/1 -> Find Max and Set Output Shift/5(Trigger)

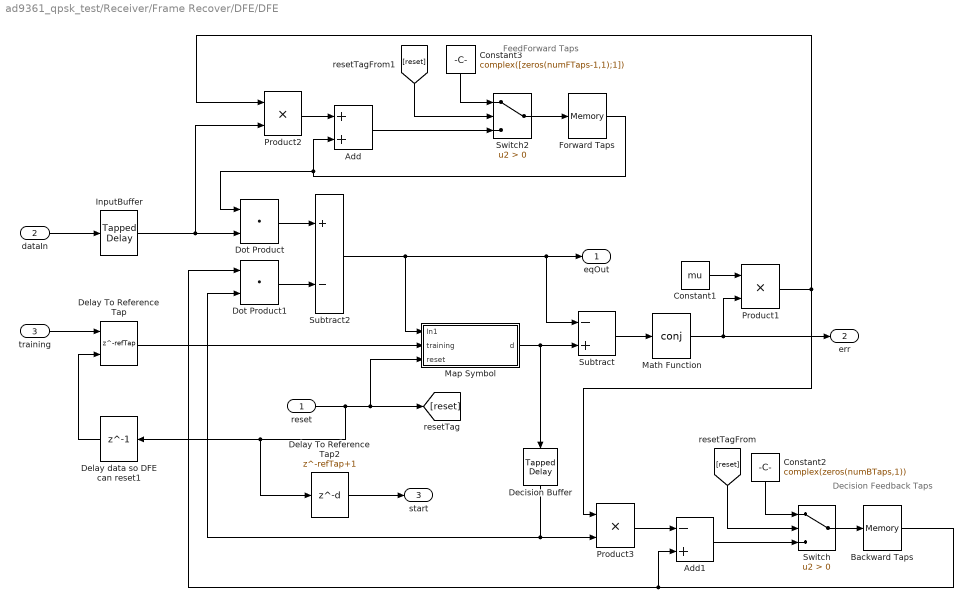
== system ad9361_qpsk_test/Receiver/Frame Recover/DFE/DFE ==
  note: FeedForward Taps
  note: Decision Feedback Taps
  reset : Inport
  dataIn : Inport  Port=2
  training : Inport  Port=3
  Add : Sum
  Add1 : Sum  Inputs=-+
  Backward Taps : Memory  InitialCondition=complex(zeros(numBTaps,1))  InheritSampleTime=on
  Constant1 : Constant  Value=mu  SampleTime=-1
  Constant2 : Constant  Value=complex(zeros(numBTaps,1))  SampleTime=-1
  Constant3 : Constant  Value=complex([zeros(numFTaps-1,1);1])  SampleTime=-1
  Decision Buffer : simulink/Discrete/Tapped Delay  vinit=0.0  samptime=-1  NumDelays=numBTaps  DelayOrder=Oldest  includeCurrent=off
  Delay To Reference Tap : Delay  DelayLength=refTap  ExternalReset=Level
      settings: InputPortMap=u0,r5
  Delay To Reference Tap2 : Delay  DelayLength=refTap+1
  Delay data so DFE can reset1 : Delay  DelayLength=1
  Dot Product : DotProduct  SaturateOnIntegerOverflow=on  InputSameDT=on  OutDataTypeStr=Inherit: Inherit via internal rule
  Dot Product1 : DotProduct  SaturateOnIntegerOverflow=on  InputSameDT=on  OutDataTypeStr=Inherit: Inherit via internal rule
  Forward Taps : Memory  InitialCondition=[complex(zeros(numFTaps-1,1));1]  InheritSampleTime=on
  InputBuffer : simulink/Discrete/Tapped Delay  vinit=0.0  samptime=-1  NumDelays=numFTaps  DelayOrder=Oldest  includeCurrent=off
  Map Symbol : Subsystem
  Math Function : Math  Operator=conj  RndMeth=Zero  SaturateOnIntegerOverflow=on
  Product1 : Product
  Product2 : Product
  Product3 : Product
  Subtract : Sum  Inputs=-+
  Subtract2 : Sum  Inputs=+-
  Switch : Switch  Criteria=u2 > Threshold
  Switch2 : Switch  Criteria=u2 > Threshold
  eqOut : Outport
  err : Outport  Port=2
  start : Outport  Port=3
  wires:
  InputBuffer/1 -> Product2/2, Dot Product/2
  Dot Product/1 -> Subtract2/1
  Dot Product1/1 -> Subtract2/2
  Subtract2/1 -> Map Symbol/1(In1), Subtract/1, eqOut/1
  Subtract/1 -> Math Function/1
  Math Function/1 -> Product1/2, err/1
  Forward Taps/1 -> Dot Product/1, Add/2
  Map Symbol/1(d) -> Subtract/2, Decision Buffer/1
  reset/1 -> Delay To Reference Tap2/1, Delay data so DFE can reset1/1, [reset], Map Symbol/3(reset)
  Constant1/1 -> Product1/1
  Backward Taps/1 -> Dot Product1/1, Add1/2
  Decision Buffer/1 -> Product3/2, Dot Product1/2
  Add1/1 -> Switch/3
  Switch/1 -> Backward Taps/1
  Constant2/1 -> Switch/1
  [reset] -> Switch/2
  Switch2/1 -> Forward Taps/1
  Add/1 -> Switch2/3
  Constant3/1 -> Switch2/1
  [reset] -> Switch2/2
  Product2/1 -> Add/1
  Product1/1 -> Product3/1, Product2/1
  Product3/1 -> Add1/1
  dataIn/1 -> InputBuffer/1
  training/1 -> Delay To Reference Tap/1
  Delay To Reference Tap/1 -> Map Symbol/2(training)
  Delay data so DFE can reset1/1 -> Delay To Reference Tap/2
  Delay To Reference Tap2/1 -> start/1

== system ad9361_qpsk_test/Receiver/Frame Recover/DFE/Packeted To Unpacked ==
  In1 : Inport
  Extract Bits : simulink/Logic and Bit Operations/Extract Bits  bitsToExtract=Range of bits  numBits=8  bitIdxRange=[1]  outScalingMode=Treat bit field as an integer
      settings: SourceProductName=Simulink
  Extract Bits1 : simulink/Logic and Bit Operations/Extract Bits  bitsToExtract=Range of bits  numBits=8  bitIdxRange=[0]  outScalingMode=Treat bit field as an integer
      settings: SourceProductName=Simulink
  Vector Concatenate : Concatenate
  Out1 : Outport
  wires:
  In1/1 -> Extract Bits1/1, Extract Bits/1
  Extract Bits/1 -> Vector Concatenate/1
  Extract Bits1/1 -> Vector Concatenate/2
  Vector Concatenate/1 -> Out1/1

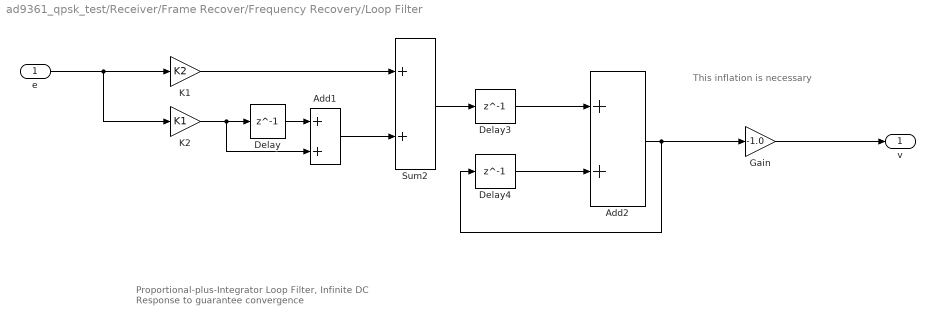
== system ad9361_qpsk_test/Receiver/Frame Recover/Frequency Recovery/Loop Filter ==
  note: This inflation is necessary
  note: Proportional-plus-Integrator Loop Filter,
      | Infinite DC Response to guarantee convergence
  e : Inport
  Add1 : Sum  RndMeth=Nearest  OutDataTypeStr=Inherit: Same as first input
  Add2 : Sum  OutDataTypeStr=Inherit: Same as first input
  Delay : Delay  DelayLength=1
  Delay3 : Delay  DelayLength=1
  Delay4 : Delay  DelayLength=1
  Gain : Gain  Gain=-1.0
  K1 : Gain  Gain=K2  OutDataTypeStr=Inherit: Same as input
  K2 : Gain  Gain=K1  OutDataTypeStr=Inherit: Same as input
  Sum2 : Sum  OutDataTypeStr=Inherit: Same as first input
  v : Outport
  wires:
  K1/1 -> Sum2/1
  Add1/1 -> Sum2/2
  e/1 -> K2/1, K1/1
  K2/1 -> Delay/1, Add1/2
  Delay/1 -> Add1/1
  Sum2/1 -> Delay3/1
  Delay3/1 -> Add2/1
  Delay4/1 -> Add2/2
  Add2/1 -> Delay4/1, Gain/1
  Gain/1 -> v/1

== system ad9361_qpsk_test/Receiver/Frame Recover/Frequency Recovery/Phase Shift FP ==
  In1 : Inport
  Phi : Inport  Port=2
  Complex Phase Shift : commutil2/Complex Phase Shift
      settings: SourceProductName=Communications Toolbox  SourceProductBaseCode=CM
  Out1 : Outport
  wires:
  Complex Phase Shift/1 -> Out1/1
  In1/1 -> Complex Phase Shift/1
  Phi/1 -> Complex Phase Shift/2

== system ad9361_qpsk_test/Receiver/Gardner Timing Recovery/Gardner TED Blocks/Imag Error ==
  data : Inport
  strobe sum : Inport  Port=2
  Delay : Delay  DelayLength=1
  Product1 : Product
  Sub : Sum  Inputs=+-
  TED Buffer Update1 : Subsystem
  Out1 : Outport
  wires:
  TED Buffer Update1/1(Middle Indx) -> Product1/1
  Delay/1 -> TED Buffer Update1/1(new data)
  TED Buffer Update1/2(oldest) -> Sub/1
  strobe sum/1 -> TED Buffer Update1/2(strobe sum)
  data/1 -> Delay/1, Sub/2
  Sub/1 -> Product1/2
  Product1/1 -> Out1/1

== system ad9361_qpsk_test/Receiver/Gardner Timing Recovery/Gardner TED Blocks/Real Error ==
  data : Inport
  strobe sum : Inport  Port=2
  Delay : Delay  DelayLength=1
  Product1 : Product
  Sub : Sum  Inputs=+-
  TED Buffer Update1 : Subsystem
  Out1 : Outport
  wires:
  TED Buffer Update1/1(Middle Indx) -> Product1/1
  Delay/1 -> TED Buffer Update1/1(new data)
  TED Buffer Update1/2(oldest) -> Sub/1
  strobe sum/1 -> TED Buffer Update1/2(strobe sum)
  data/1 -> Delay/1, Sub/2
  Sub/1 -> Product1/2
  Product1/1 -> Out1/1

== system ad9361_qpsk_test/Receiver/Gardner Timing Recovery/InterpControl_Blocks/Calculate New mu ==
  W : Inport
  NCOCounter : Inport  Port=2
  Math Reciprocal : Math  Operator=reciprocal  OutDataTypeStr=Inherit: Inherit via back propagation  RndMeth=Zero  SaturateOnIntegerOverflow=on
  Product : Product  OutDataTypeStr=Inherit: Inherit via back propagation
  mu : Outport
  wires:
  W/1 -> Math Reciprocal/1
  NCOCounter/1 -> Product/2
  Math Reciprocal/1 -> Product/1
  Product/1 -> mu/1

== system ad9361_qpsk_test/Receiver/Gardner Timing Recovery/InterpControl_Blocks/Mod 1 ==
  In1 : Inport
  Add : Sum
  Compare To Constant : simulink/Logic and Bit Operations/Compare To Constant  relop=<  const=1  OutDataTypeStr=boolean
  Compare To Constant1 : simulink/Logic and Bit Operations/Compare To Constant  relop=>=  const=0  OutDataTypeStr=boolean
  Constant : Constant  OutDataTypeStr=fixdt(0,1,0)  SampleTime=-1
  Constant1 : Constant  OutDataTypeStr=fixdt(0,1,0)  SampleTime=-1
  Logical Operator : Logic  AllPortsSameDT=off  OutDataTypeStr=boolean
  Subtract : Sum  Inputs=+-
  Switch : Switch  Criteria=u2 > Threshold
  Switch1 : Switch
  Out1 : Outport
  wires:
  Logical Operator/1 -> Switch/2
  Compare To Constant/1 -> Logical Operator/2
  Compare To Constant1/1 -> Logical Operator/1
  In1/1 -> Subtract/1, Add/1, Switch/1, Compare To Constant/1, Compare To Constant1/1, Switch1/2
  Add/1 -> Switch1/3
  Subtract/1 -> Switch1/1
  Switch1/1 -> Switch/3
  Constant1/1 -> Add/2
  Constant/1 -> Subtract/2
  Switch/1 -> Out1/1

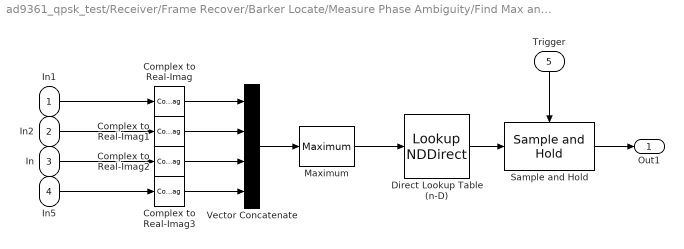
== system ad9361_qpsk_test/Receiver/Frame Recover/Barker Locate/Measure Phase Ambiguity/Find Max and Set Output Shift ==
  In1 : Inport
  In2 : Inport  Port=2
  In : Inport  Port=3
  In5 : Inport  Port=4
  Trigger : Inport  Port=5
  Complex to Real-Imag{,1..3} (4 alike) : ComplexToRealImag  Output=Imag
  Direct Lookup Table (n-D) : LookupNDDirect  NumberOfTableDimensions=1  Table=exp(-(0:pi/2:(pi*3/2)) .* 1i).'  DiagnosticForOutOfRangeInput=Error
  Maximum : dspstat3/Maximum  operation=maximum  fcn=Index  indexBase=Zero  operateOver=Each column  Dimension=1  InputProcessing=Columns as channels (frame based)  reset=None  roiEnable=off  roiType=Rectangles  roiPortion=Entire ROI  roiOutput=Individual statistics for each ROI  roiFlag=off  roundingMode=Floor  overflowMode=off  accumDataTypeStr=Inherit: Same as product output  accumLastDataTypeStr=Inherit: Same as product output
  Sample and Hold : dspsigops/Sample and Hold  trig=Rising edge  initCond=1  latchinput=off
  Vector Concatenate : Concatenate  NumInputs=4
  Out1 : Outport
  wires:
  In/1 -> Complex to Real-Imag2/1
  Vector Concatenate/1 -> Maximum/1
  Direct Lookup Table (n-D)/1 -> Sample and Hold/1
  In1/1 -> Complex to Real-Imag/1
  Sample and Hold/1 -> Out1/1
  Trigger/1 -> Sample and Hold/Trigger
  Complex to Real-Imag2/1 -> Vector Concatenate/3
  Complex to Real-Imag1/1 -> Vector Concatenate/2
  In5/1 -> Complex to Real-Imag3/1
  Complex to Real-Imag3/1 -> Vector Concatenate/4
  Complex to Real-Imag/1 -> Vector Concatenate/1
  Maximum/1 -> Direct Lookup Table (n-D)/1
  In2/1 -> Complex to Real-Imag1/1

== system ad9361_qpsk_test/Receiver/Frame Recover/DFE/DFE/Map Symbol ==
  In1 : Inport
  training : Inport  Port=2
  reset : Inport  Port=3
  Decision Directed : Subsystem
  Delay : Delay  DelayLength=1
  HDL Counter : hdlsllib/Sources/HDL Counter  CountType=Count limited  CountInit=0  CountStep=1  CountMax=2^18  CountFromType=Initial value  CountFrom=0  CountResetPort=on  CountLoadPort=off  CountEnbPort=off  CountDirPort=off  CountDataType=Unsigned  CountWordLen=32  CountFracLen=0  CountSampTime=1
      settings: SourceProductBaseCode=HD
  Switch : Switch  Criteria=u2 > Threshold  Threshold=numTrainingSamples
  d : Outport
  wires:
  In1/1 -> Decision Directed/1(eqOut)
  Switch/1 -> d/1
  reset/1 -> HDL Counter/1
  HDL Counter/1 -> Switch/2
  Decision Directed/1(decision) -> Switch/1
  training/1 -> Delay/1
  Delay/1 -> Switch/3

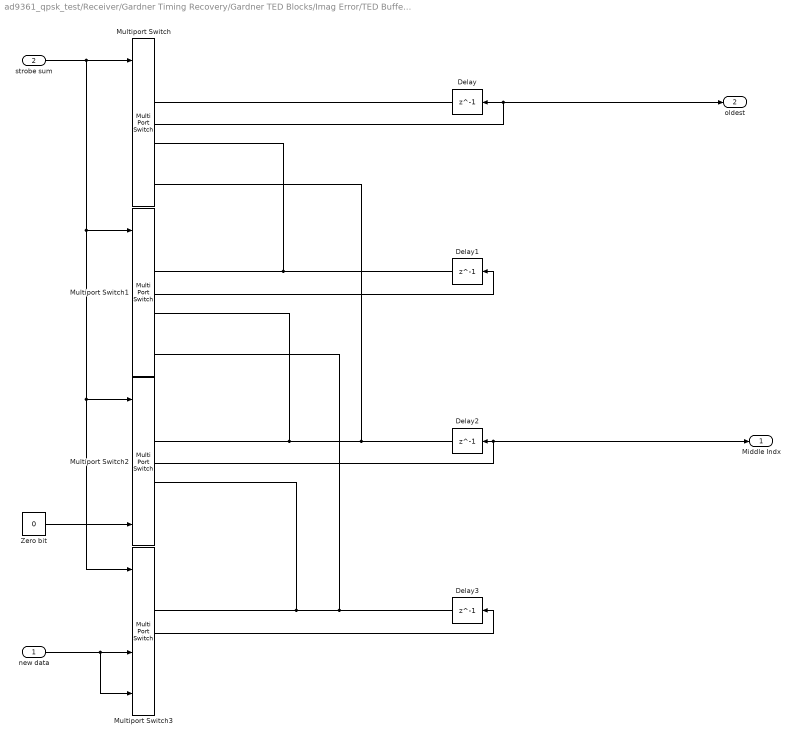
== system ad9361_qpsk_test/Receiver/Gardner Timing Recovery/Gardner TED Blocks/Imag Error/TED Buffer Update1 ==
  new data : Inport
  strobe sum : Inport  Port=2
  Delay{,1..3} (4 alike) : Delay  DelayLength=1
  Multiport Switch{,1..3} (4 alike) : MultiPortSwitch  DataPortOrder=Zero-based contiguous  DataPortIndices={0,1,[2,3]}  zeroidx=on
  Zero bit : Constant  Value=0  SampleTime=1/RadioSampleRate
  Middle Indx : Outport
  oldest : Outport  Port=2
  wires:
  Multiport Switch/1 -> oldest/1, Delay/1
  Multiport Switch3/1 -> Delay3/1
  Multiport Switch2/1 -> Delay2/1, Middle Indx/1
  Multiport Switch1/1 -> Delay1/1
  Delay3/1 -> Multiport Switch3/2, Multiport Switch2/3, Multiport Switch1/4
  Zero bit/1 -> Multiport Switch2/4
  new data/1 -> Multiport Switch3/3, Multiport Switch3/4
  Delay2/1 -> Multiport Switch2/2, Multiport Switch1/3, Multiport Switch/4
  Delay1/1 -> Multiport Switch1/2, Multiport Switch/3
  Delay/1 -> Multiport Switch/2
  strobe sum/1 -> Multiport Switch/1, Multiport Switch1/1, Multiport Switch2/1, Multiport Switch3/1

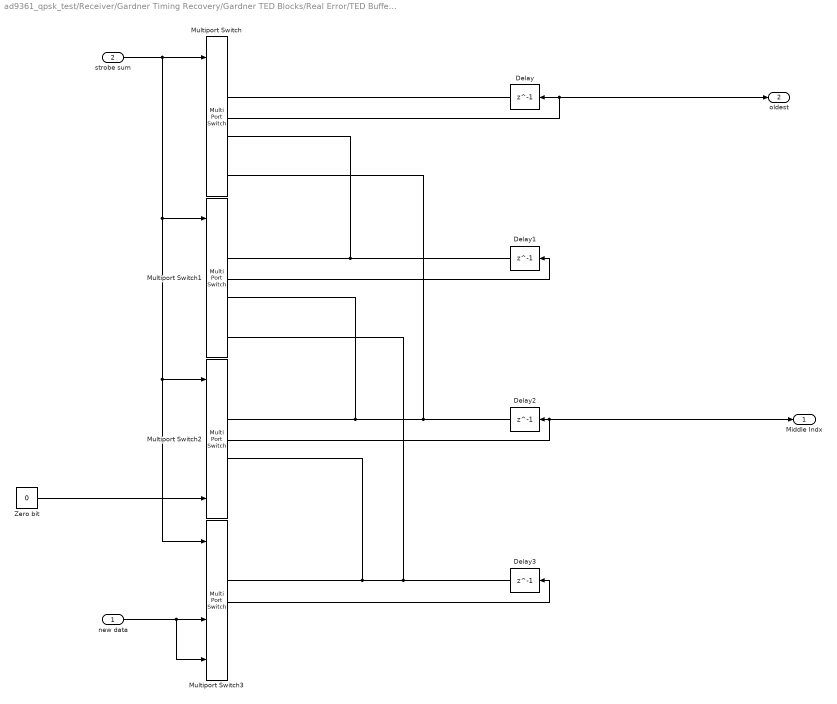
== system ad9361_qpsk_test/Receiver/Gardner Timing Recovery/Gardner TED Blocks/Real Error/TED Buffer Update1 ==
  new data : Inport
  strobe sum : Inport  Port=2
  Delay{,1..3} (4 alike) : Delay  DelayLength=1
  Multiport Switch{,1..3} (4 alike) : MultiPortSwitch  DataPortOrder=Zero-based contiguous  DataPortIndices={0,1,[2,3]}  zeroidx=on
  Zero bit : Constant  Value=0  SampleTime=1/RadioSampleRate
  Middle Indx : Outport
  oldest : Outport  Port=2
  wires:
  Multiport Switch/1 -> oldest/1, Delay/1
  Multiport Switch3/1 -> Delay3/1
  Multiport Switch2/1 -> Delay2/1, Middle Indx/1
  Multiport Switch1/1 -> Delay1/1
  Delay3/1 -> Multiport Switch3/2, Multiport Switch2/3, Multiport Switch1/4
  new data/1 -> Multiport Switch3/3, Multiport Switch3/4
  Delay2/1 -> Multiport Switch2/2, Multiport Switch1/3, Multiport Switch/4
  Delay1/1 -> Multiport Switch1/2, Multiport Switch/3
  Delay/1 -> Multiport Switch/2
  strobe sum/1 -> Multiport Switch/1, Multiport Switch1/1, Multiport Switch2/1, Multiport Switch3/1
  Zero bit/1 -> Multiport Switch2/4

== system ad9361_qpsk_test/Receiver/Frame Recover/DFE/DFE/Map Symbol/Decision Directed ==
  eqOut : Inport
  Compare To Zero : simulink/Logic and Bit Operations/Compare To Zero  relop=>=  OutDataTypeStr=boolean
  Compare To Zero1 : simulink/Logic and Bit Operations/Compare To Zero  relop=>=  OutDataTypeStr=boolean
  Complex to Real-Imag : ComplexToRealImag
  QPSK Decisions : LookupNDDirect  Table=[-0.7071 - 0.7071i, -0.7071 + 0.7071i; 0.7071 - 0.7071i, 0.7071 + 0.7071i]  DiagnosticForOutOfRangeInput=Error
  decision : Outport
  wires:
  eqOut/1 -> Complex to Real-Imag/1
  Complex to Real-Imag/1 -> Compare To Zero/1
  Complex to Real-Imag/2 -> Compare To Zero1/1
  Compare To Zero/1 -> QPSK Decisions/1
  Compare To Zero1/1 -> QPSK Decisions/2
  QPSK Decisions/1 -> decision/1

== matlab function ad9361_qpsk_test/Receiver/Frame Recover/Frequency Recovery/PED ==
  data: In input; e output
function e  = PED(In)


e = sign(real(In)).*imag(In) - sign(imag(In)).*real(In);
